simulink model "V1_Pendel_Validierung"  (R2022a)
settings: Solver=ode3  StartTime=0.0  StopTime=Zeit(end)  FixedStep=0.001  RelTol=1e-3
values from neighbouring files (symbols this model uses):
  d = 0.0035    [V1_Parameter_Stahl_math.m]    (also in V1_Parameter_Stahl_phys.m = 0.0036; V1_Parameter_Styropor_math.m = 0.0001771; V1_Parameter_Styropor_phys.m = 0.0016)
  g = 9.81    [V1_Parameter_Stahl_math.m]    (also in V1_Parameter_Stahl_phys.m; V1_Parameter_Styropor_math.m; V1_Parameter_Styropor_phys.m)
  J = m * (l.^2)    [V1_Parameter_Stahl_math.m]    (also in V1_Parameter_Stahl_phys.m = J_A + J_SA + J_KA; V1_Parameter_Styropor_math.m; V1_Parameter_Styropor_phys.m = J_A + J_SA + J_KA)
  l = l_s - s + r_k    (= 0.600875)    [V1_Parameter_Stahl_math.m]    (also in V1_Parameter_Stahl_phys.m = 0.459624859903; V1_Parameter_Styropor_math.m = 0.6004; V1_Parameter_Styropor_phys.m = 0.0522377280265)
  m = 1.396    [V1_Parameter_Stahl_math.m]    (also in V1_Parameter_Stahl_phys.m = 1.8737; V1_Parameter_Styropor_math.m = 0.0047; V1_Parameter_Styropor_phys.m = 0.4824)
  phi_0_rad = phi_0 * (pi/180)    [V1_Parameter_Stahl_math.m]    (also in V1_Parameter_Stahl_phys.m; V1_Parameter_Styropor_math.m; V1_Parameter_Styropor_phys.m)
settings Model: Creator=bornk  LastModifiedBy=bornk

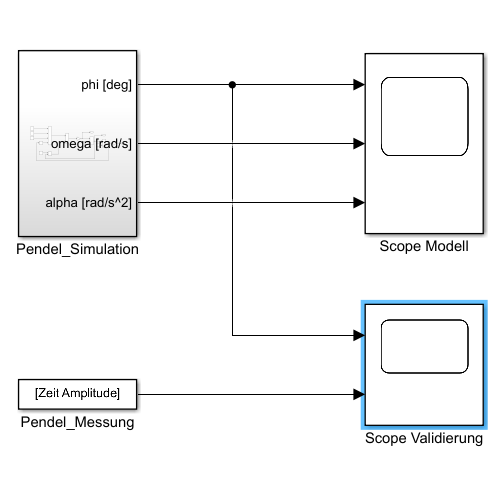
[thumbnail: Simulink's stored preview of the top-level diagram]
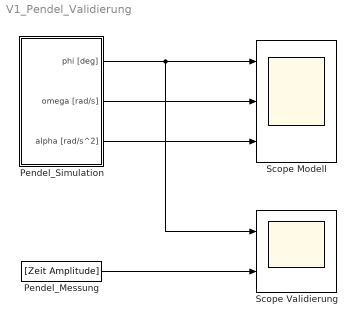
== system V1_Pendel_Validierung ==
  Pendel_Messung : FromWorkspace  VariableName=[Zeit Amplitude]
  Pendel_Simulation : Subsystem
  Scope Modell : Scope  NumInputPorts=3
  Scope Validierung : Scope  NumInputPorts=2
  wires:
  Pendel_Simulation/2(omega [rad/s]) -> Scope Modell/2
  Pendel_Simulation/3(alpha [rad/s^2]) -> Scope Modell/3
  Pendel_Simulation/1(phi [deg]) -> Scope Validierung/1, Scope Modell/1
  Pendel_Messung/1 -> Scope Validierung/2

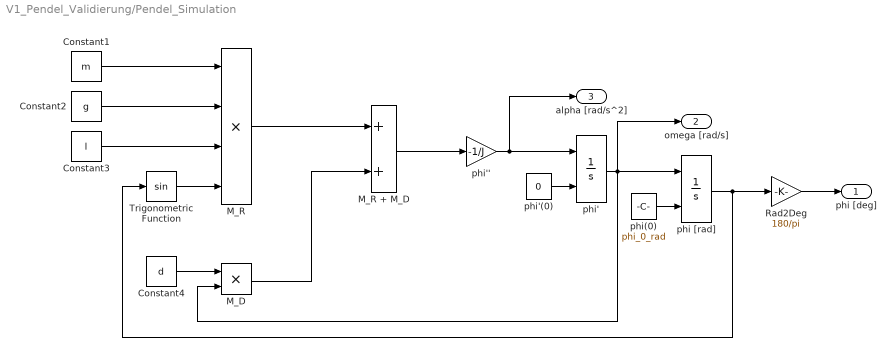
== system V1_Pendel_Validierung/Pendel_Simulation ==
  Constant1 : Constant  Value=m
  Constant2 : Constant  Value=g
  Constant3 : Constant  Value=l
  Constant4 : Constant  Value=d
  M_D : Product
  M_R : Product  Inputs=4
  M_R + M_D : Sum
  Rad2Deg : Gain  Gain=180/pi
  Trigonometric Function : Trigonometry
  phi [rad] : Integrator  InitialConditionSource=external
  phi' : Integrator  InitialConditionSource=external
  phi'' : Gain  Gain=-1/J
  phi'(0) : Constant  Value=0
  phi(0) : Constant  Value=phi_0_rad
  phi [deg] : Outport
  omega [rad/s] : Outport  Port=2
  alpha [rad/s^2] : Outport  Port=3
  wires:
  M_R/1 -> M_R + M_D/1
  Constant2/1 -> M_R/2
  Constant1/1 -> M_R/1
  phi'(0)/1 -> phi'/2
  Constant4/1 -> M_D/1
  phi'/1 -> omega [rad/s]/1, phi [rad]/1, M_D/2
  phi(0)/1 -> phi [rad]/2
  M_D/1 -> M_R + M_D/2
  Trigonometric Function/1 -> M_R/4
  M_R + M_D/1 -> phi''/1
  Constant3/1 -> M_R/3
  phi [rad]/1 -> Trigonometric Function/1, Rad2Deg/1
  phi''/1 -> alpha [rad/s^2]/1, phi'/1
  Rad2Deg/1 -> phi [deg]/1
